simulink model "practica2armax"  (Simulink 5.0)
settings: Solver=ode45  StartTime=0.0  StopTime=7000  RelTol=1e-3
undefined symbols (not defined in the file): ts
libraries: simulink x19, dspstat3 x4, dsparch3 x1, dsparch4 x1
settings Model: LastModifiedBy=pc1  BlockReductionOpt=off  BooleanDataType=off

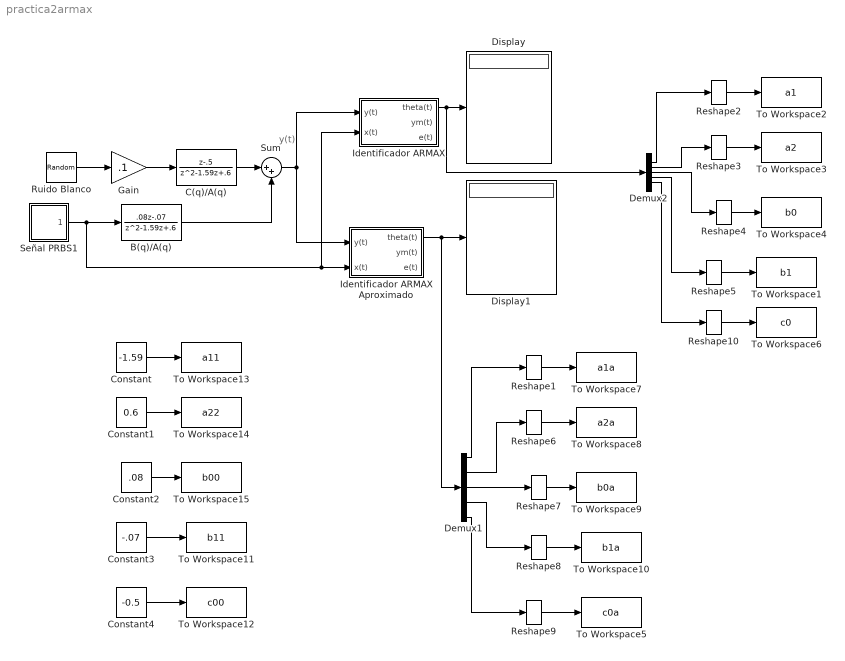
== system practica2armax ==
  note: y(t)
  B(q)/A(q) : DiscreteTransferFcn  Numerator=[.08 -.07]  Denominator=[1 -1.59 .6]  SampleTime=ts
  C(q)/A(q) : DiscreteTransferFcn  Numerator=[1 -.5]  Denominator=[1 -1.59 .6]  SampleTime=ts
  Constant : Constant  Value=-1.59
  Constant1 : Constant  Value=0.6
  Constant2 : Constant  Value=.08
  Constant3 : Constant  Value=-.07
  Constant4 : Constant  Value=-0.5
  Demux1 : Demux  Outputs=5
  Demux2 : Demux  Outputs=5
  Display : Display
  Display1 : Display
  Gain : Gain  Gain=.1  SaturateOnIntegerOverflow=on
  Identificador ARMAX : Subsystem  mask(rolo){l=0.01, ts=ts, nk=0, na=2, nb=2, nc=1}
      mask prompts: l "valor landa"; ts "valor ts"; nk "valor nk"; na "Valor na"; nb "valor nb"; nc "valor nc"
  Identificador ARMAX Aproximado : Subsystem  mask(rolo){s=.1, ts=ts, nk=0, na=2, nb=2, nc=1}
      mask prompts: s "valor de s"; ts "valor ts"; nk "valor nk"; na "Valor na"; nb "valor nb"; nc "valor nc"
  Reshape{1..10} (10 alike) : simulink/Math Operations/Reshape  OutputDimensionality=1-D array  OutputDimensions=[1,1]
  Ruido Blanco : RandomNumber  Variance=.1  SampleTime=0
  Señal PRBS1 : Subsystem
  Sum : Sum  Inputs=|++  SaturateOnIntegerOverflow=on  InputSameDT=on
  To Workspace1 : ToWorkspace  VariableName=b1  SampleTime=-1  SaveFormat=Array
  To Workspace10 : ToWorkspace  VariableName=b1a  SampleTime=-1  SaveFormat=Array
  To Workspace11 : ToWorkspace  VariableName=b11  SampleTime=-1  SaveFormat=Array
  To Workspace12 : ToWorkspace  VariableName=c00  SampleTime=-1  SaveFormat=Array
  To Workspace13 : ToWorkspace  VariableName=a11  SampleTime=-1  SaveFormat=Array
  To Workspace14 : ToWorkspace  VariableName=a22  SampleTime=-1  SaveFormat=Array
  To Workspace15 : ToWorkspace  VariableName=b00  SampleTime=-1  SaveFormat=Array
  To Workspace2 : ToWorkspace  VariableName=a1  SampleTime=-1  SaveFormat=Array
  To Workspace3 : ToWorkspace  VariableName=a2  SampleTime=-1  SaveFormat=Array
  To Workspace4 : ToWorkspace  VariableName=b0  SampleTime=-1  SaveFormat=Array
  To Workspace5 : ToWorkspace  VariableName=c0a  SampleTime=-1  SaveFormat=Array
  To Workspace6 : ToWorkspace  VariableName=c0  SampleTime=-1  SaveFormat=Array
  To Workspace7 : ToWorkspace  VariableName=a1a  SampleTime=-1  SaveFormat=Array
  To Workspace8 : ToWorkspace  VariableName=a2a  SampleTime=-1  SaveFormat=Array
  To Workspace9 : ToWorkspace  VariableName=b0a  SampleTime=-1  SaveFormat=Array
  wires:
  C(q)/A(q)/1 -> Sum/1
  B(q)/A(q)/1 -> Sum/2
  Señal PRBS1/1(u ( t )) -> B(q)/A(q)/1, Identificador ARMAX Aproximado/2(x(t)), Identificador ARMAX/2(x(t))
  Ruido Blanco/1 -> Gain/1
  Identificador ARMAX Aproximado/1(theta(t)) -> Display1/1, Demux1/1
  Sum/1 -> Identificador ARMAX Aproximado/1(y(t)), Identificador ARMAX/1(y(t))
  Gain/1 -> C(q)/A(q)/1
  Identificador ARMAX/1(theta(t)) -> Display/1, Demux2/1
  Demux1/1 -> Reshape1/1
  Demux1/2 -> Reshape6/1
  Demux1/3 -> Reshape7/1
  Demux1/4 -> Reshape8/1
  Reshape1/1 -> To Workspace7/1
  Reshape6/1 -> To Workspace8/1
  Reshape7/1 -> To Workspace9/1
  Reshape8/1 -> To Workspace10/1
  Demux2/1 -> Reshape2/1
  Demux2/2 -> Reshape3/1
  Demux2/3 -> Reshape4/1
  Demux2/4 -> Reshape5/1
  Reshape2/1 -> To Workspace2/1
  Reshape3/1 -> To Workspace3/1
  Reshape4/1 -> To Workspace4/1
  Reshape5/1 -> To Workspace1/1
  Reshape9/1 -> To Workspace5/1
  Demux1/5 -> Reshape9/1
  Reshape10/1 -> To Workspace6/1
  Demux2/5 -> Reshape10/1
  Constant/1 -> To Workspace13/1
  Constant1/1 -> To Workspace14/1
  Constant2/1 -> To Workspace15/1
  Constant3/1 -> To Workspace11/1
  Constant4/1 -> To Workspace12/1

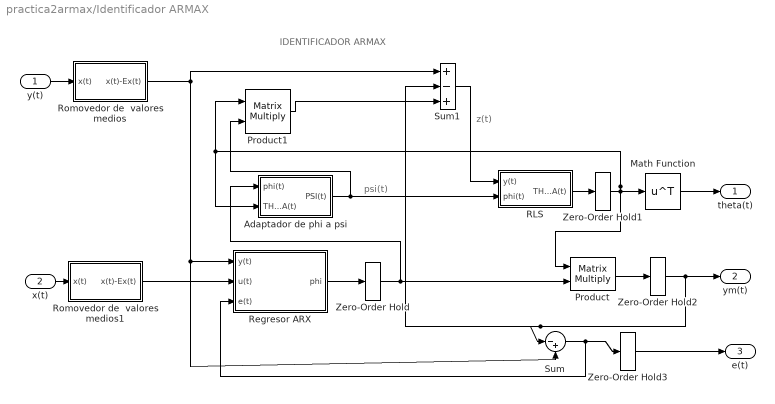
== system practica2armax/Identificador ARMAX ==
  note: psi(t)
  note: IDENTIFICADOR ARMAX
  note: z(t)
  y(t) : Inport
  x(t) : Inport  Port=2
  Adaptador de phi a psi : Subsystem
  Math Function : Math  Operator=transpose
  Product : Product  Multiplication=Matrix(*)  SaturateOnIntegerOverflow=on  InputSameDT=on
  Product1 : Product  Multiplication=Matrix(*)  SaturateOnIntegerOverflow=on  InputSameDT=on
  RLS : Subsystem
  Regresor ARX : Subsystem
  Romovedor de  valores medios : Subsystem
  Romovedor de  valores medios1 : Subsystem
  Sum : Sum  Inputs=|-+  SaturateOnIntegerOverflow=on  InputSameDT=on
  Sum1 : Sum  Inputs=|+-+  SaturateOnIntegerOverflow=on  InputSameDT=on
  Zero-Order Hold{,1..3} (4 alike) : ZeroOrderHold  SampleTime=ts
  theta(t) : Outport
  ym(t) : Outport  Port=2
  e(t) : Outport  Port=3
  wires:
  Sum1/1 -> RLS/1(y(t))
  Product1/1 -> Sum1/3
  Adaptador de phi a psi/1(PSI(t)) -> Product1/2, RLS/2(phi(t))
  Zero-Order Hold3/1 -> e(t)/1
  Sum/1 -> Regresor ARX/3(e(t)), Zero-Order Hold3/1
  Zero-Order Hold2/1 -> Sum1/2, Sum/1, ym(t)/1
  Product/1 -> Zero-Order Hold2/1
  Zero-Order Hold1/1 -> Product/1, Adaptador de phi a psi/2(THETA(t)), Product1/1, Math Function/1
  Zero-Order Hold/1 -> Adaptador de phi a psi/1(phi(t)), Product/2
  RLS/1(THETA(t)) -> Zero-Order Hold1/1
  x(t)/1 -> Romovedor de  valores medios1/1(x(t))
  y(t)/1 -> Romovedor de  valores medios/1(x(t))
  Romovedor de  valores medios/1(x(t)-Ex(t)) -> Sum1/1, Sum/2, Regresor ARX/1(y(t))
  Romovedor de  valores medios1/1(x(t)-Ex(t)) -> Regresor ARX/2(u(t))
  Regresor ARX/1(phi) -> Zero-Order Hold/1
  Math Function/1 -> theta(t)/1

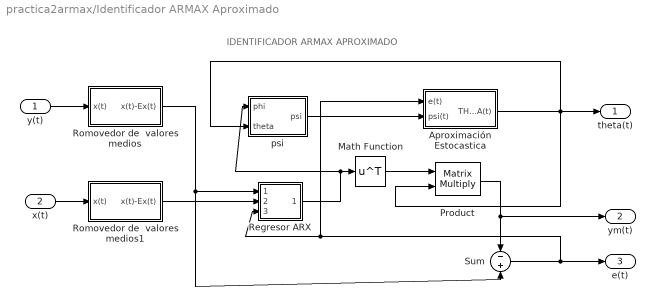
== system practica2armax/Identificador ARMAX Aproximado ==
  note: IDENTIFICADOR ARMAX APROXIMADO
  y(t) : Inport
  x(t) : Inport  Port=2
  Aproximación Estocastica : Subsystem
  Math Function : Math  Operator=transpose
  Product : Product  Multiplication=Matrix(*)  SaturateOnIntegerOverflow=on  InputSameDT=on
  Regresor ARX : Subsystem
  Romovedor de  valores medios : Subsystem
  Romovedor de  valores medios1 : Subsystem
  Sum : Sum  Inputs=-+  SaturateOnIntegerOverflow=on  InputSameDT=on
  psi : Subsystem
  theta(t) : Outport
  ym(t) : Outport  Port=2
  e(t) : Outport  Port=3
  wires:
  psi/1(psi) -> Aproximación Estocastica/2(psi(t))
  Math Function/1 -> Product/1
  Sum/1 -> e(t)/1, Regresor ARX/3(e(t)), Aproximación Estocastica/1(e(t))
  Product/1 -> ym(t)/1, Sum/1
  Aproximación Estocastica/1(THETA(t)) -> Product/2, theta(t)/1, psi/2(theta)
  x(t)/1 -> Romovedor de  valores medios1/1(x(t))
  y(t)/1 -> Romovedor de  valores medios/1(x(t))
  Romovedor de  valores medios/1(x(t)-Ex(t)) -> Sum/2, Regresor ARX/1(y(t))
  Regresor ARX/1(phi) -> Math Function/1, psi/1(phi)
  Romovedor de  valores medios1/1(x(t)-Ex(t)) -> Regresor ARX/2(u(t))

== system practica2armax/Señal PRBS1 ==
  Random Number : RandomNumber  Variance=.1  SampleTime=0
  Sign : Signum
  Zero-Order Hold : ZeroOrderHold  SampleTime=ts
  u ( t ) : Outport
  wires:
  Zero-Order Hold/1 -> u ( t )/1
  Sign/1 -> Zero-Order Hold/1
  Random Number/1 -> Sign/1

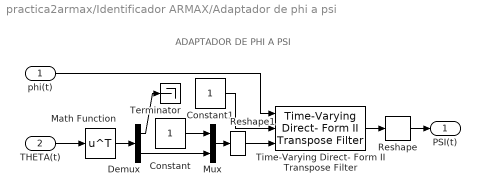
== system practica2armax/Identificador ARMAX/Adaptador de phi a psi ==
  note: ADAPTADOR DE PHI A PSI
  phi(t) : Inport
  THETA(t) : Inport  Port=2
  Constant : Constant
  Constant1 : Constant
  Demux : Demux  Outputs=[na+nb,nc]
  Math Function : Math  Operator=transpose
  Mux : Mux  Inputs=2
  Reshape : simulink/Math Operations/Reshape  OutputDimensionality=Column vector  OutputDimensions=[1,1]
  Reshape1 : simulink/Math Operations/Reshape  OutputDimensionality=Column vector  OutputDimensions=[1,1]
  Terminator : Terminator
  Time-Varying Direct- Form II Transpose Filter : dsparch3/Time-Varying Direct- Form II Transpose Filter  NumDen=Pole-Zero (IIR)  ic=0  filtCheck=on  FiltPerFrame=One Filter Per Frame Time
  PSI(t) : Outport
  wires:
  Time-Varying Direct- Form II Transpose Filter/1 -> Reshape/1
  Demux/1 -> Terminator/1
  phi(t)/1 -> Time-Varying Direct- Form II Transpose Filter/1
  Constant1/1 -> Time-Varying Direct- Form II Transpose Filter/2
  Constant/1 -> Mux/1
  Demux/2 -> Mux/2
  THETA(t)/1 -> Math Function/1
  Reshape/1 -> PSI(t)/1
  Math Function/1 -> Demux/1
  Mux/1 -> Reshape1/1
  Reshape1/1 -> Time-Varying Direct- Form II Transpose Filter/3

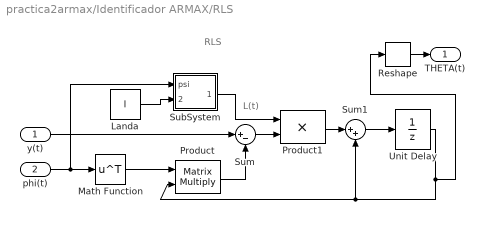
== system practica2armax/Identificador ARMAX/RLS ==
  note: L(t)
  note: RLS
  y(t) : Inport
  phi(t) : Inport  Port=2
  Landa : Constant  Value=l
  Math Function : Math  Operator=transpose
  Product : Product  Multiplication=Matrix(*)  SaturateOnIntegerOverflow=on  InputSameDT=on
  Product1 : Product  SaturateOnIntegerOverflow=on  InputSameDT=on
  Reshape : simulink/Math Operations/Reshape  OutputDimensionality=Row vector  OutputDimensions=[1,1]
  SubSystem : Subsystem
  Sum : Sum  Inputs=|+-  SaturateOnIntegerOverflow=on  InputSameDT=on
  Sum1 : Sum  Inputs=|++  SaturateOnIntegerOverflow=on  InputSameDT=on
  Unit Delay : UnitDelay  X0=zeros(1,na+nb+nc)'  SampleTime=ts
  THETA(t) : Outport
  wires:
  phi(t)/1 -> SubSystem/1(psi), Math Function/1
  Math Function/1 -> Product/1
  Unit Delay/1 -> Product/2, Sum1/2, Reshape/1
  Product/1 -> Sum/2
  y(t)/1 -> Sum/1
  Sum/1 -> Product1/2
  SubSystem/1(L(t)) -> Product1/1
  Landa/1 -> SubSystem/2(landa)
  Sum1/1 -> Unit Delay/1
  Product1/1 -> Sum1/1
  Reshape/1 -> THETA(t)/1

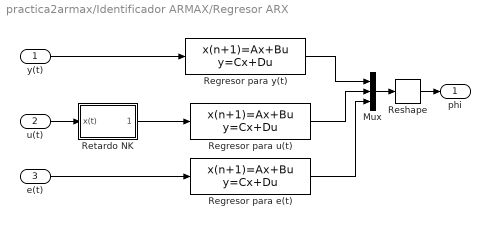
== system practica2armax/Identificador ARMAX/Regresor ARX ==
  y(t) : Inport
  u(t) : Inport  Port=2
  e(t) : Inport  Port=3
  Mux : Mux  Inputs=3
  Regresor para e(t) : DiscreteStateSpace  A=[zeros(1,nc);eye(nc-1,nc)]  B=[1,zeros(1,nc-1)]'  C=eye(nc)  D=[zeros(nc,1)]  SampleTime=ts
  Regresor para u(t) : DiscreteStateSpace  A=[zeros(1,nb);eye(nb-1,nb)]  B=[1,zeros(1,nb-1)]'  C=eye(nb)  D=[zeros(nb,1)]  SampleTime=ts
  Regresor para y(t) : DiscreteStateSpace  A=[zeros(1,na);eye(na-1,na)]  B=[-1,zeros(1,na-1)]'  C=eye(na)  D=[zeros(na,1)]  SampleTime=ts
  Reshape : simulink/Math Operations/Reshape  OutputDimensionality=Column vector  OutputDimensions=[1,1]
  Retardo NK : Subsystem  mask{nk=0}
      mask prompts: nk "Valor nk"
  phi : Outport
  wires:
  Regresor para e(t)/1 -> Mux/3
  e(t)/1 -> Regresor para e(t)/1
  Retardo NK/1(x(t-nk)) -> Regresor para u(t)/1
  u(t)/1 -> Retardo NK/1(x(t))
  Mux/1 -> Reshape/1
  y(t)/1 -> Regresor para y(t)/1
  Regresor para u(t)/1 -> Mux/2
  Regresor para y(t)/1 -> Mux/1
  Reshape/1 -> phi/1

== system practica2armax/Identificador ARMAX/Romovedor de  valores medios ==
  x(t) : Inport
  Mean : dspstat3/Mean  run=on  reset_popup=None
  Sum : Sum  Inputs=|-+  SaturateOnIntegerOverflow=on  InputSameDT=on
  Zero-Order Hold : ZeroOrderHold  SampleTime=ts
  x(t)-Ex(t) : Outport
  wires:
  x(t)/1 -> Zero-Order Hold/1
  Zero-Order Hold/1 -> Mean/1, Sum/2
  Mean/1 -> Sum/1
  Sum/1 -> x(t)-Ex(t)/1

== system practica2armax/Identificador ARMAX/Romovedor de  valores medios1 ==
  x(t) : Inport
  Mean : dspstat3/Mean  run=on  reset_popup=None
  Sum : Sum  Inputs=|-+  SaturateOnIntegerOverflow=on  InputSameDT=on
  Zero-Order Hold : ZeroOrderHold  SampleTime=ts
  x(t)-Ex(t) : Outport
  wires:
  x(t)/1 -> Zero-Order Hold/1
  Zero-Order Hold/1 -> Mean/1, Sum/2
  Mean/1 -> Sum/1
  Sum/1 -> x(t)-Ex(t)/1

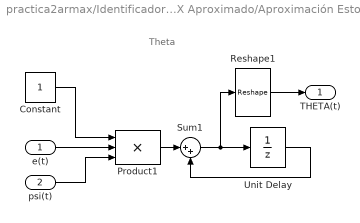
== system practica2armax/Identificador ARMAX Aproximado/Aproximación Estocastica ==
  note: Theta
  e(t) : Inport
  psi(t) : Inport  Port=2
  Constant : Constant
  Product1 : Product  Inputs=3  SaturateOnIntegerOverflow=on  InputSameDT=on
  Reshape1 : simulink/Math Operations/Reshape  OutputDimensionality=Column vector  OutputDimensions=[1,1]
  Sum1 : Sum  Inputs=|++  SaturateOnIntegerOverflow=on  InputSameDT=on
  Unit Delay : UnitDelay  X0=zeros(1,na+nb+nc)'  SampleTime=ts
  THETA(t) : Outport
  wires:
  Unit Delay/1 -> Sum1/2
  Sum1/1 -> Unit Delay/1, Reshape1/1
  Reshape1/1 -> THETA(t)/1
  Constant/1 -> Product1/1
  e(t)/1 -> Product1/2
  psi(t)/1 -> Product1/3
  Product1/1 -> Sum1/1

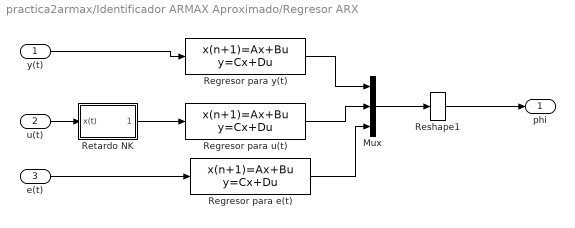
== system practica2armax/Identificador ARMAX Aproximado/Regresor ARX ==
  y(t) : Inport
  u(t) : Inport  Port=2
  e(t) : Inport  Port=3
  Mux : Mux  Inputs=[na nb nc]
  Regresor para e(t) : DiscreteStateSpace  A=[zeros(1,nc);eye(nc-1,nc)]  B=[1,zeros(1,nc-1)]'  C=eye(nc)  D=[zeros(nc,1)]  SampleTime=ts
  Regresor para u(t) : DiscreteStateSpace  A=[zeros(1,nb);eye(nb-1,nb)]  B=[1,zeros(1,nb-1)]'  C=eye(nb)  D=[zeros(nb,1)]  SampleTime=ts
  Regresor para y(t) : DiscreteStateSpace  A=[zeros(1,na);eye(na-1,na)]  B=[-1,zeros(1,na-1)]'  C=eye(na)  D=[zeros(na,1)]  SampleTime=ts
  Reshape1 : simulink/Math Operations/Reshape  OutputDimensionality=Column vector  OutputDimensions=[1,1]
  Retardo NK : Subsystem  mask{nk=0}
      mask prompts: nk "Valor nk"
  phi : Outport
  wires:
  Regresor para e(t)/1 -> Mux/3
  e(t)/1 -> Regresor para e(t)/1
  Retardo NK/1(x(t-nk)) -> Regresor para u(t)/1
  u(t)/1 -> Retardo NK/1(x(t))
  y(t)/1 -> Regresor para y(t)/1
  Regresor para u(t)/1 -> Mux/2
  Regresor para y(t)/1 -> Mux/1
  Reshape1/1 -> phi/1
  Mux/1 -> Reshape1/1

== system practica2armax/Identificador ARMAX Aproximado/Romovedor de  valores medios ==
  x(t) : Inport
  Mean : dspstat3/Mean  run=on  reset_popup=None
  Sum : Sum  Inputs=|-+  SaturateOnIntegerOverflow=on  InputSameDT=on
  Zero-Order Hold : ZeroOrderHold  SampleTime=ts
  x(t)-Ex(t) : Outport
  wires:
  x(t)/1 -> Zero-Order Hold/1
  Zero-Order Hold/1 -> Mean/1, Sum/2
  Mean/1 -> Sum/1
  Sum/1 -> x(t)-Ex(t)/1

== system practica2armax/Identificador ARMAX Aproximado/Romovedor de  valores medios1 ==
  x(t) : Inport
  Mean : dspstat3/Mean  run=on  reset_popup=None
  Sum : Sum  Inputs=|-+  SaturateOnIntegerOverflow=on  InputSameDT=on
  Zero-Order Hold : ZeroOrderHold  SampleTime=ts
  x(t)-Ex(t) : Outport
  wires:
  x(t)/1 -> Zero-Order Hold/1
  Zero-Order Hold/1 -> Mean/1, Sum/2
  Mean/1 -> Sum/1
  Sum/1 -> x(t)-Ex(t)/1

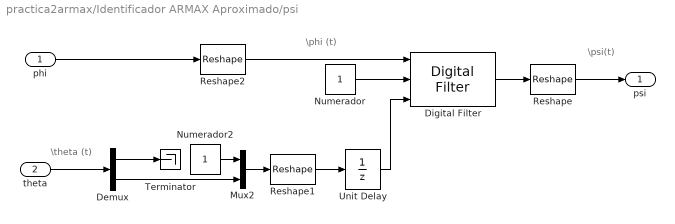
== system practica2armax/Identificador ARMAX Aproximado/psi ==
  note: \phi (t)
  note: \psi(t)
  note: \theta (t)
  phi : Inport
  theta : Inport  Port=2
  Demux : Demux  Outputs=[na+nb nc]
  Digital Filter : dsparch4/Digital Filter  TypePopup=IIR (poles & zeros)  IIRFiltStruct=Direct form I  AllPoleFiltStruct=Direct form  FIRFiltStruct=Direct form  CoeffSource=Input port(s)  NumCoeffs=[1 2]  DenCoeffs=[1 0.1]  BiQuadCoeffs=[1 0.3 0.4 1 0.1 0.2]  LatticeCoeffs=[0.2 0.4]  denIgnore=on  FiltPerSampPopup=One filter per frame  IC=0  ICnum=0  ICden=0
  Mux2 : Mux  Inputs=2
  Numerador : Constant
  Numerador2 : Constant
  Reshape : simulink/Math Operations/Reshape  OutputDimensionality=Column vector  OutputDimensions=[1,1]
  Reshape1 : simulink/Math Operations/Reshape  OutputDimensionality=Row vector  OutputDimensions=[1,3]
  Reshape2 : simulink/Math Operations/Reshape  OutputDimensionality=Row vector  OutputDimensions=[1,3]
  Terminator : Terminator
  Unit Delay : UnitDelay
  psi : Outport
  wires:
  Digital Filter/1 -> Reshape/1
  theta/1 -> Demux/1
  Numerador/1 -> Digital Filter/2
  Demux/1 -> Terminator/1
  Reshape/1 -> psi/1
  Numerador2/1 -> Mux2/1
  Demux/2 -> Mux2/2
  Mux2/1 -> Reshape1/1
  Reshape2/1 -> Digital Filter/1
  phi/1 -> Reshape2/1
  Reshape1/1 -> Unit Delay/1
  Unit Delay/1 -> Digital Filter/3

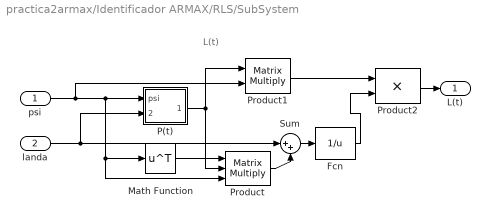
== system practica2armax/Identificador ARMAX/RLS/SubSystem ==
  note: L(t)
  psi : Inport
  landa : Inport  Port=2
  Fcn : Fcn  Expr=1/u
  Math Function : Math  Operator=transpose
  P(t) : Subsystem
  Product : Product  Inputs=3  Multiplication=Matrix(*)  SaturateOnIntegerOverflow=on  InputSameDT=on
  Product1 : Product  Multiplication=Matrix(*)  SaturateOnIntegerOverflow=on  InputSameDT=on
  Product2 : Product  SaturateOnIntegerOverflow=on  InputSameDT=on
  Sum : Sum  Inputs=|++  SaturateOnIntegerOverflow=on  InputSameDT=on
  L(t) : Outport
  wires:
  Product2/1 -> L(t)/1
  psi/1 -> P(t)/1(psi), Math Function/1, Product/3, Product1/2
  landa/1 -> P(t)/2(landa), Sum/1
  Math Function/1 -> Product/1
  Product/1 -> Sum/2
  Sum/1 -> Fcn/1
  Fcn/1 -> Product2/2
  Product1/1 -> Product2/1
  P(t)/1(P(t-1)) -> Product/2, Product1/1

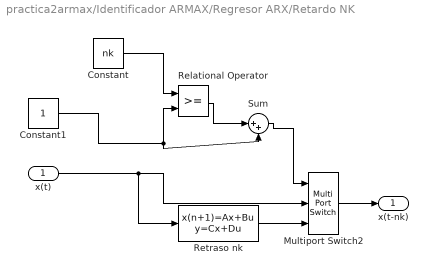
== system practica2armax/Identificador ARMAX/Regresor ARX/Retardo NK ==
  x(t) : Inport
  Constant : Constant  Value=nk
  Constant1 : Constant
  Multiport Switch2 : MultiPortSwitch  Inputs=2  SaturateOnIntegerOverflow=on  InputSameDT=on
  Relational Operator : RelationalOperator  InputSameDT=on
  Retraso nk : DiscreteStateSpace  A=[zeros(1,max(nk,1));eye(max(nk,1)-1,max(nk,1))]  B=[1,zeros(1,max(nk,1)-1)]'  C=[zeros(1,max(nk,1)-1),1]  D=[0]  SampleTime=ts
  Sum : Sum  Inputs=|++  SaturateOnIntegerOverflow=on  InputSameDT=on
  x(t-nk) : Outport
  wires:
  x(t)/1 -> Retraso nk/1, Multiport Switch2/2
  Multiport Switch2/1 -> x(t-nk)/1
  Retraso nk/1 -> Multiport Switch2/3
  Sum/1 -> Multiport Switch2/1
  Relational Operator/1 -> Sum/1
  Constant/1 -> Relational Operator/1
  Constant1/1 -> Sum/2, Relational Operator/2

== system practica2armax/Identificador ARMAX Aproximado/Regresor ARX/Retardo NK ==
  x(t) : Inport
  Constant : Constant  Value=nk
  Constant1 : Constant
  Multiport Switch2 : MultiPortSwitch  Inputs=2  SaturateOnIntegerOverflow=on  InputSameDT=on
  Relational Operator : RelationalOperator  InputSameDT=on
  Retraso nk : DiscreteStateSpace  A=[zeros(1,max(nk,1));eye(max(nk,1)-1,max(nk,1))]  B=[1,zeros(1,max(nk,1)-1)]'  C=[zeros(1,max(nk,1)-1),1]  D=[0]  SampleTime=ts
  Sum : Sum  Inputs=|++  SaturateOnIntegerOverflow=on  InputSameDT=on
  x(t-nk) : Outport
  wires:
  x(t)/1 -> Retraso nk/1, Multiport Switch2/2
  Multiport Switch2/1 -> x(t-nk)/1
  Retraso nk/1 -> Multiport Switch2/3
  Sum/1 -> Multiport Switch2/1
  Relational Operator/1 -> Sum/1
  Constant/1 -> Relational Operator/1
  Constant1/1 -> Sum/2, Relational Operator/2

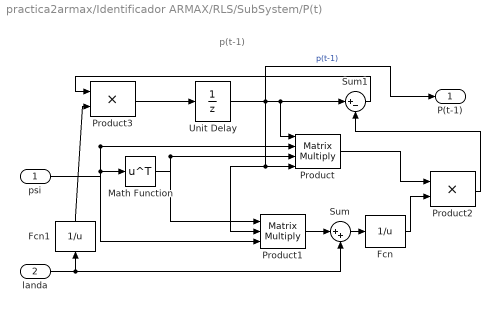
== system practica2armax/Identificador ARMAX/RLS/SubSystem/P(t) ==
  note: p(t-1)
  psi : Inport
  landa : Inport  Port=2
  Fcn : Fcn  Expr=1/u
  Fcn1 : Fcn  Orientation=up  Expr=1/u
  Math Function : Math  Operator=transpose
  Product : Product  Inputs=4  Multiplication=Matrix(*)  SaturateOnIntegerOverflow=on  InputSameDT=on
  Product1 : Product  Inputs=3  Multiplication=Matrix(*)  SaturateOnIntegerOverflow=on  InputSameDT=on
  Product2 : Product  SaturateOnIntegerOverflow=on  InputSameDT=on
  Product3 : Product  SaturateOnIntegerOverflow=on  InputSameDT=on
  Sum : Sum  Inputs=|++  SaturateOnIntegerOverflow=on  InputSameDT=on
  Sum1 : Sum  Inputs=|+-  SaturateOnIntegerOverflow=on  InputSameDT=on
  Unit Delay : UnitDelay  X0=100000*eye(na+nb+nc)  SampleTime=ts
  P(t-1) : Outport
  wires:
  Fcn1/1 -> Product3/2
  psi/1 -> Math Function/1, Product/2, Product1/3
  Unit Delay/1 -> Product/4, Product1/2, Product/1, Sum1/1, P(t-1)/1  "p(t-1)"
  Math Function/1 -> Product/3, Product1/1
  Product1/1 -> Sum/1
  landa/1 -> Fcn1/1, Sum/2
  Sum/1 -> Fcn/1
  Fcn/1 -> Product2/2
  Product/1 -> Product2/1
  Product2/1 -> Sum1/2
  Sum1/1 -> Product3/1
  Product3/1 -> Unit Delay/1
